simulink model "PubIfDecisionTOS_MDL"  (R2020b)
settings: configuration reference "DspaceConfig" (kept outside this file)
PostLoadFcn:
  | if any(exist('dsrtsu_mdlpostloadfcn', 'file') ~= 0), dsrtsu_mdlpostloadfcn('Execute', bdroot); end
InitFcn:
  | , if any(exist('dsmpb_private', 'file') ~= 0), dsmpb_private('dsmpb_mdlclblib', 'Init', bdroot); end,
undefined symbols (not defined in the file or in its folder): C_TOS_ACCEgoRAxletoFbumplength_m, C_TOS_ACCTargetFront_Flag, C_TOS_AEBJAPedObjDxThre_Val, C_TOS_AEBJAPedObjDyThre_Val, C_TOS_AEBJATargetSize_Val, C_TOS_AEBJAVehObjDxThre_Val, C_TOS_AEBJAVehObjDyThre_Val, C_TOS_AEBJuncPedTargetSize_Val, C_TOS_AEBLatObjDxThre_Val, C_TOS_AEBLatPedDyThre_Val, C_TOS_AEBLatTargetSize_Val, C_TOS_AEBLongTargetInEgoFront_Flag, C_TOS_axAbsGround_Parameter, C_TOS_CameraConfirmedFlag, C_TOS_CNsubjWidth, C_TOS_CurrentLaneCoreMinWidth_Val, C_TOS_CutInProb_Val_Zero, C_TOS_CutOutProb_Val_Zero, C_TOS_D2R_Val, C_TOS_DefaultValueObjectToCenterLine_dy, C_TOS_EgoCarWidth_Val, C_TOS_EgoDxRefPoint_m, C_TOS_EgoRAxletoFbumplength_m, C_TOS_HalfWidthVehicle_Con, C_TOS_HWA_CurrentLaneFlag, C_TOS_HWA_LeftLaneFlag, C_TOS_HWA_MovingDir_Vaild, C_TOS_HWA_MovState_Vaild, C_TOS_HWA_RightLaneFlag, C_TOS_LaneLineCourseErrorFront, C_TOS_LaneLineCourseErrorRear, C_TOS_MotorbikeDefaultWidth_m, C_TOS_NumberOfEffectiveTargets, C_TOS_Obj_Age_Val, C_TOS_Objdx_Constraint_Val, C_TOS_ObjectDefaultWidth_m, C_TOS_ObjInCurrentLane_Val, C_TOS_ObjInCurrentLaneValid, C_TOS_ObjInLeftLaneValid, C_TOS_ObjInRightLaneValid, C_TOS_ObjNotInCurrentLane_Val, C_TOS_ObjNotREElementType, C_TOS_ObjPredictDis_dy_ConstantVal_Zeros, C_TOS_ObjToCenterLine_ConstantVal_Zeros, C_TOS_OFMObjIDInvilad_Val, C_TOS_PIL_LatDisCons_Val_zero, C_TOS_PIL_ObjectCutInFlag_b, C_TOS_PIL_ObjectCutOutFlag_b, C_TOS_PIL_ObjLaneProb_al_Val, C_TOS_PP_ObjFusType_FC_Confirm_b, C_TOS_PP_ObjFusType_FC_FR_Confirm_b, C_TOS_PP_ObjFusType_FR_Confirm_b, C_TOS_RE_80BoolDefault_Val, C_TOS_RE_80Single181Default_Val, C_TOS_RE_80Single255Default_Val, C_TOS_RE_80Uint8Default_Val, C_TOS_RE_D2R, C_TOS_RE_D_180_Val, C_TOS_RE_InvalidObjectID_Val, C_TOS_RE_InvalidTargetChainDir_Val ... (+142)
libraries: simulink x1650, TOS_LIB x361, canfdmsglib x14
(part 51 of 69)

== system PubIfDecisionTOS_MDL/TOS_20201112/TOS_2012080320/TOS/ACC/TOS_ACCCurrentLane/ACC_CurrentLane_Target/TOS_ACC_P0/ACC_P0_Targe/ACC_P0_Targe/TOS_ACC_ObstacleProbConfirm/TOS_ACCObstacleProbAborDly ==
  ACC_Target_ID_K1 : Inport
  ObjectID : Inport  Port=2
  TOS_ACCObstacleProb : Inport  Port=3
  If : If  IfExpression=u1
  If Action Subsystem : Subsystem  TreatAsAtomicUnit=on
  If Action Subsystem1 : Subsystem  TreatAsAtomicUnit=on
  Merge : Merge
  Subsystem : Subsystem
  TOS_ACCObstacleProbFilt : Outport
  wires:
  If/1 -> If Action Subsystem1/Action
  TOS_ACCObstacleProb/1 -> If Action Subsystem1/1(TOS_ACCFusionType), If Action Subsystem/1(TOS_ACCFusionType)
  If/2 -> If Action Subsystem/Action
  ACC_Target_ID_K1/1 -> Subsystem/1(ACC_TargetP0_ID_K1)
  ObjectID/1 -> Subsystem/2(ObjectID)
  Subsystem/1(ACC_SameTargetP0) -> If/1
  If Action Subsystem1/1(TOS_ACCFusionTypeFilt) -> Merge/1
  If Action Subsystem/1(TOS_ACCFusionTypeFilt) -> Merge/2
  Merge/1 -> TOS_ACCObstacleProbFilt/1

== system PubIfDecisionTOS_MDL/TOS_20201112/TOS_2012080320/TOS/ACC/TOS_ACCCurrentLane/ACC_CurrentLane_Target/TOS_ACC_P0/ACC_P0_Targe/ACC_P0_Targe/TOS_ACC_TargetMovingDirConfirm/Subsystem ==
  ObjMovState : Inport
  ACC_Target_ID_K1 : Inport  Port=2
  ACC_Target_ID_K2 : Inport  Port=3
  ACC_Target_MovState_K1 : Inport  Port=4
  ACC_Target_MovState_K2 : Inport  Port=5
  ObjectID : Inport  Port=6
  TOS_ObjMovStateCfmFlow : Stateflow chart  TreatAsAtomicUnit=on
  TOS_ObjMovStateCfm : Outport
  wires:
  TOS_ObjMovStateCfmFlow/1(TOS_ObjMovStateCfm) -> TOS_ObjMovStateCfm/1
  ACC_Target_ID_K1/1 -> TOS_ObjMovStateCfmFlow/1(Target_ID_K1)
  ACC_Target_ID_K2/1 -> TOS_ObjMovStateCfmFlow/2(Target_ID_K2)
  ACC_Target_MovState_K1/1 -> TOS_ObjMovStateCfmFlow/3(Target_MovState_K1)
  ACC_Target_MovState_K2/1 -> TOS_ObjMovStateCfmFlow/4(Target_MovState_K2)
  ObjMovState/1 -> TOS_ObjMovStateCfmFlow/5(ObjMovState)
  ObjectID/1 -> TOS_ObjMovStateCfmFlow/6(ObjectID)

== system PubIfDecisionTOS_MDL/TOS_20201112/TOS_2012080320/TOS/ACC/TOS_ACCCurrentLane/ACC_CurrentLane_Target/TOS_ACC_P0/ACC_P0_Targe/ACC_P0_Targe/TOS_ACC_TargetMovingDirConfirm/TOS_ACCMovingDirAborDly ==
  ACC_TargetP0_ID_K1 : Inport
  ObjectID : Inport  Port=2
  TOS_ACCMovingDir : Inport  Port=3
  If : If  IfExpression=u1
  If Action Subsystem : Subsystem  TreatAsAtomicUnit=on
  If Action Subsystem1 : Subsystem  TreatAsAtomicUnit=on
  Merge : Merge
  Subsystem : Subsystem
  TOS_ACC_TrgMovDirFlag_6_ObserVale : Outport
  TOS_ACC_TrgMovDir : Outport  Port=2
  wires:
  If/1 -> If Action Subsystem1/Action
  TOS_ACCMovingDir/1 -> If Action Subsystem1/1(TOS_ACCMovingDir), If Action Subsystem/1(TOS_ACCMovingDir)
  If/2 -> If Action Subsystem/Action
  ACC_TargetP0_ID_K1/1 -> Subsystem/1(ACC_TargetP0_ID_K1)
  ObjectID/1 -> Subsystem/2(ObjectID)
  Subsystem/1(ACC_SameTargetP0) -> TOS_ACC_TrgMovDirFlag_6_ObserVale/1, If/1
  If Action Subsystem1/1(TOS_ACCMovingDirFilt) -> Merge/1
  If Action Subsystem/1(TOS_ACCMovingDirFilt) -> Merge/2
  Merge/1 -> TOS_ACC_TrgMovDir/1

== system PubIfDecisionTOS_MDL/TOS_20201112/TOS_2012080320/TOS/ACC/TOS_ACCCurrentLane/ACC_CurrentLane_Target/TOS_ACC_P0/ACC_P0_Targe/ACC_P0_Targe/TOS_ACC_TargetMovingDirConfirm/TOS_ACC_TargetMovingDirConfirm_V2011170316(备份) ==
  note: 已选中目标，前两个周期为运动，以后为运动，前两个周期为Stopped，以后为Stopped
  note: 去除横穿目标
  object_MovingState : Inport
  PP_ObjMovingDirSignalProcessing : Inport  Port=2
  Object_HeadingAngle : Inport  Port=3
  Object_VX : Inport  Port=4
  Object_VY : Inport  Port=5
  VIE_EgoVelocity : Inport  Port=6
  SteerWheelAng : Inport  Port=7
  ACC_Target_ID_K1 : Inport  Port=8
  ACC_Target_ID_K2 : Inport  Port=9
  ACC_Target_MovState_K1 : Inport  Port=10
  ACC_Target_MovState_K2 : Inport  Port=11
  ObjectID : Inport  Port=12
  Abs{,1..4} (5 alike) : Abs
  Add : Sum
  Compare To Constant : simulink/Logic and Bit Operations/Compare To Constant  relop===  const=ObjectMovingOrientation_E.SameDir  OutDataTypeStr=boolean
      settings: AttributesFormatString=ObjectMovingOrientation_E.SameDir = 1
  Compare To Constant1 : simulink/Logic and Bit Operations/Compare To Constant  relop===  const=OFM_OBJ_MOVINGSTATE_E.MOVING  OutDataTypeStr=boolean
      settings: AttributesFormatString=OFM_OBJ_MOVINGSTATE_E.MOVING = 2
  Compare To Constant10 : simulink/Logic and Bit Operations/Compare To Constant  relop=<=  const=P_TOS_ObjLatCroYawAngMaxThre_Val  OutDataTypeStr=boolean
      settings: AttributesFormatString=P_TOS_ObjLatCroYawAngMaxThre_Val = 135
  Compare To Constant11 : simulink/Logic and Bit Operations/Compare To Constant  relop===  const=1  OutDataTypeStr=boolean
  Compare To Constant12 : simulink/Logic and Bit Operations/Compare To Constant  relop===  const=2  OutDataTypeStr=boolean
  Compare To Constant13 : simulink/Logic and Bit Operations/Compare To Constant  relop=<  const=1.5  OutDataTypeStr=boolean
      settings: AttributesFormatString=1.5 m/s
  Compare To Constant2 : simulink/Logic and Bit Operations/Compare To Constant  relop=>=  const=P_TOS_ObjInSameDirYawAngMinThre_Val  OutDataTypeStr=boolean
      settings: AttributesFormatString=P_TOS_ObjInSameDirYawAngMinThre_Val = 0
  Compare To Constant3 : simulink/Logic and Bit Operations/Compare To Constant  relop=<=  const=P_TOS_ObjInSameDirYawAngMaxThre_Val  OutDataTypeStr=boolean
      settings: AttributesFormatString=P_TOS_ObjInSameDirYawAngMaxThre_Val = 45
  Compare To Constant4 : simulink/Logic and Bit Operations/Compare To Constant  relop===  const=OFM_OBJ_MOVINGSTATE_E.MOVING_SLOWLY  OutDataTypeStr=boolean
      settings: AttributesFormatString=OFM_OBJ_MOVINGSTATE_E.MOVING_SLOWLY = 5
  Compare To Constant5 : simulink/Logic and Bit Operations/Compare To Constant  relop=<  const=P_TOS_SameDirVyOffset_Val  OutDataTypeStr=boolean
      settings: AttributesFormatString=P_TOS_SameDirVyOffset_Val = 2
  Compare To Constant6 : simulink/Logic and Bit Operations/Compare To Constant  relop===  const=ObjectMovingOrientation_E.Crossing  OutDataTypeStr=boolean
      settings: AttributesFormatString=ObjectMovingOrientation_E.Crossing = 3
  Compare To Constant7 : simulink/Logic and Bit Operations/Compare To Constant  relop=>=  const=P_TOS_LongVyThre_Val  OutDataTypeStr=boolean
      settings: AttributesFormatString=P_TOS_LongVyThre_Val = 2
  Compare To Constant8 : simulink/Logic and Bit Operations/Compare To Constant  relop===  const=OFM_OBJ_MOVINGSTATE_E.STOPPED  OutDataTypeStr=boolean
      settings: AttributesFormatString=OFM_OBJ_MOVINGSTATE_E.STOPPED = 4
  Compare To Constant9 : simulink/Logic and Bit Operations/Compare To Constant  relop=>=  const=P_TOS_ObjInSameDirYawAngMaxThre_Val  OutDataTypeStr=boolean
      settings: AttributesFormatString=P_TOS_ObjInSameDirYawAngMaxThre_Val = 45
  Constant1 : Constant  Value=P_TOS_SameDirVxvOffset_Val
      settings: AttributesFormatString=P_TOS_AEBLong_SameDirVxvOffset_Val = 1
  Constant2 : Constant  Value=0  OutDataTypeStr=boolean
  Constant3 : Constant  OutDataTypeStr=boolean
  Constant4 : Constant  OutDataTypeStr=boolean
  Data Type Conversion1 : DataTypeConversion  OutDataTypeStr=Enum: ObjectMovingOrientation_E
  Data Type Conversion2 : DataTypeConversion  OutDataTypeStr=Enum: OFM_OBJ_MOVINGSTATE_E
  Logical Operator{,3,6,8} (4 alike) : Logic  AllPortsSameDT=off  OutDataTypeStr=boolean
  Logical Operator{1,4..5,7} (4 alike) : Logic  Operator=OR  AllPortsSameDT=off  OutDataTypeStr=boolean
  Logical Operator2 : Logic  Operator=OR  Inputs=3  AllPortsSameDT=off  OutDataTypeStr=boolean
  Relational Operator : RelationalOperator  Operator=<  OutDataTypeStr=boolean  RndMeth=Simplest
  Subsystem : Subsystem
  Switch : Switch  Criteria=u2 > Threshold
  Switch1 : Switch  Criteria=u2 ~= 0
  Switch2 : Switch  Criteria=u2 ~= 0
  TOS_ACCMovingDirAborDly : Subsystem
  Terminator : Terminator
  Terminator1 : Terminator
  TOS_ACC_TrgMovDir : Outport
  TOS_ACC_TrgMovDirFlag_1_ObserVale : Outport  Port=2
  TOS_ACC_TrgMovDirFlag_2_ObserVale : Outport  Port=3
  TOS_ACC_TrgMovDirFlag_3_ObserVale : Outport  Port=4
  TOS_ACC_TrgMovDirFlag_4_ObserVale : Outport  Port=5
  TOS_ACC_TrgMovDirFlag_5_ObserVale : Outport  Port=6
  TOS_ACC_TrgMovDirFlag_6_ObserVale : Outport  Port=7
  wires:
  Compare To Constant13/1 -> Logical Operator8/2
  Abs3/1 -> Compare To Constant13/1
  [Object_VY] -> Abs3/1
  Constant4/1 -> Logical Operator8/1
  TOS_ACCMovingDirAborDly/2(TOS_ACC_TrgMovDir) -> TOS_ACC_TrgMovDir/1
  TOS_ACCMovingDirAborDly/1(TOS_ACC_TrgMovDirFlag_6_ObserVale) -> [TOS_ACC_TrgMovDirFlag_6_ObserVale]
  [TOS_ACC_TrgMovDirFlag_6_ObserVale] -> TOS_ACC_TrgMovDirFlag_6_ObserVale/1
  [TOS_ACC_TrgMovDirFlag_5_ObserVale] -> TOS_ACC_TrgMovDirFlag_5_ObserVale/1
  [TOS_ACC_TrgMovDirFlag_4_ObserVale] -> TOS_ACC_TrgMovDirFlag_4_ObserVale/1
  [TOS_ACC_TrgMovDirFlag_3_ObserVale] -> TOS_ACC_TrgMovDirFlag_3_ObserVale/1
  [TOS_ACC_TrgMovDirFlag_2_ObserVale] -> TOS_ACC_TrgMovDirFlag_2_ObserVale/1
  [TOS_ACC_TrgMovDirFlag_1_ObserVale] -> TOS_ACC_TrgMovDirFlag_1_ObserVale/1
  Logical Operator7/1 -> Switch2/2, [TOS_ACC_TrgMovDirFlag_3_ObserVale]
  Compare To Constant12/1 -> Logical Operator7/1
  ACC_Target_ID_K1/1 -> Subsystem/2(ACC_Target_ID_K1), [ACC_Target_ID_K1]
  ACC_Target_MovState_K1/1 -> Subsystem/4(ACC_Target_MovState_K1)
  ACC_Target_ID_K2/1 -> Subsystem/3(ACC_Target_ID_K2)
  ACC_Target_MovState_K2/1 -> Subsystem/5(ACC_Target_MovState_K2)
  Data Type Conversion2/1 -> Compare To Constant4/1, Subsystem/1(ObjMovState), Compare To Constant8/1, Compare To Constant1/1
  Subsystem/1(TOS_ObjMovStateCfm) -> Compare To Constant12/1, Compare To Constant11/1
  Compare To Constant11/1 -> Logical Operator2/3
  ObjectID/1 -> Subsystem/6(ObjectID), [ObjectID]
  Logical Operator8/1 -> Switch2/1
  Switch2/1 -> Switch/3
  Compare To Constant8/1 -> Logical Operator7/2
  Switch1/1 -> Switch2/3
  Logical Operator6/1 -> Logical Operator5/2
  Compare To Constant10/1 -> Logical Operator6/2
  Compare To Constant9/1 -> Logical Operator6/1
  [Object_HeadingAngle] -> Compare To Constant9/1, Compare To Constant10/1
  Compare To Constant6/1 -> Logical Operator5/1
  [PP_ObjMovingDirSignalProcessing] -> Compare To Constant6/1
  Switch/1 -> TOS_ACCMovingDirAborDly/3(TOS_ACCMovingDir), [TOS_ACC_TrgMovDirFlag_5_ObserVale]
  [ObjectID] -> TOS_ACCMovingDirAborDly/2(ObjectID)
  [ACC_Target_ID_K1] -> TOS_ACCMovingDirAborDly/1(ACC_TargetP0_ID_K1)
  Abs4/1 -> Compare To Constant7/1
  [Object_VY] -> Abs4/1
  Logical Operator5/1 -> Logical Operator4/1
  Compare To Constant7/1 -> Logical Operator4/2
  Constant2/1 -> Switch1/1
  Logical Operator4/1 -> Switch1/2, [TOS_ACC_TrgMovDirFlag_4_ObserVale]
  Constant3/1 -> Switch1/3
  SteerWheelAng/1 -> Terminator/1
  Abs2/1 -> Compare To Constant5/1
  Object_VY/1 -> Abs2/1, [Object_VY]
  Object_VX/1 -> Abs1/1
  VIE_EgoVelocity/1 -> Relational Operator/2
  Add/1 -> Relational Operator/1
  Constant1/1 -> Add/2
  Abs1/1 -> Add/1
  Relational Operator/1 -> Logical Operator/1
  Compare To Constant5/1 -> Logical Operator/2
  Logical Operator/1 -> Logical Operator1/2
  Abs/1 -> [Object_HeadingAngle], Compare To Constant3/1, Compare To Constant2/1
  PP_ObjMovingDirSignalProcessing/1 -> Data Type Conversion1/1
  Logical Operator1/1 -> [TOS_ACC_TrgMovDirFlag_1_ObserVale], Switch/1
  Data Type Conversion1/1 -> [PP_ObjMovingDirSignalProcessing], Compare To Constant/1
  Compare To Constant2/1 -> Logical Operator3/1
  Compare To Constant3/1 -> Logical Operator3/2
  Object_HeadingAngle/1 -> Abs/1
  Compare To Constant/1 -> Logical Operator1/1
  Logical Operator3/1 -> Terminator1/1
  object_MovingState/1 -> Data Type Conversion2/1
  Compare To Constant4/1 -> Logical Operator2/2
  Compare To Constant1/1 -> Logical Operator2/1
  Logical Operator2/1 -> Switch/2, [TOS_ACC_TrgMovDirFlag_2_ObserVale]

== system PubIfDecisionTOS_MDL/TOS_20201112/TOS_2012080320/TOS/ACC/TOS_ACCCurrentLane/ACC_CurrentLane_Target/TOS_ACC_P1/ACC_P1_Targe/ACC_P1_Targe/TOS_ACC_DyConfirm/OverLapConfirm ==
  DyConfirm_Sig : Inport
  Abs{,1..4} (5 alike) : Abs
  Bus Creator{1..4} (4 alike) : BusCreator  Inputs=2
  Bus Selector : BusSelector  OutputSignals=PositionFlag,Line_pC2
  Bus Selector1 : BusSelector  OutputSignals=PositionFlag,Line_pC2
  Bus Selector2 : BusSelector  OutputSignals=LM_LR_Line04_pC0,LM_RL_Line04_pC0
  Bus Selector3 : BusSelector  OutputSignals=PositionFlag,Line_pC2
  Bus Selector4 : BusSelector  OutputSignals=LM_LR_Line04_pC2,Object_DX,LM_LR_Line04_dDisStart,LM_LR_Line04_dDisEnd,LM_LR_Line04_fCamValid
  Bus Selector5 : BusSelector  OutputSignals=LM_LR_Line05_pC2,Object_DX,LM_LR_Line05_dDisStart,LM_LR_Line05_dDisEnd,LM_LR_Line05_fCamValid
  Bus Selector8 : BusSelector  OutputSignals=LM_LR_Line06_pC2,Object_DX,LM_LR_Line06_dDisStart,LM_LR_Line06_dDisEnd,LM_LR_Line06_fCamValid
  Compare To Constant : simulink/Logic and Bit Operations/Compare To Constant  relop===  const=uint8(4)  OutDataTypeStr=boolean
  Compare To Constant1 : simulink/Logic and Bit Operations/Compare To Constant  relop=>=  const=single(0.001)  OutDataTypeStr=boolean
  Compare To Constant2 : simulink/Logic and Bit Operations/Compare To Constant  relop=>=  const=single(0.001)  OutDataTypeStr=boolean
  Compare To Constant3 : simulink/Logic and Bit Operations/Compare To Constant  relop===  const=uint8(5)  OutDataTypeStr=boolean
  Compare To Constant4 : simulink/Logic and Bit Operations/Compare To Constant  relop=>=  const=single(0.001)  OutDataTypeStr=boolean
  Compare To Constant5 : simulink/Logic and Bit Operations/Compare To Constant  relop===  const=uint8(6)  OutDataTypeStr=boolean
  Constant : Constant  Value=0  OutDataTypeStr=uint8
  Constant1 : Constant  Value=4  OutDataTypeStr=uint8
  Constant2 : Constant  Value=5  OutDataTypeStr=uint8
  Constant3 : Constant  Value=6  OutDataTypeStr=uint8
  Constant4 : Constant  Value=0  OutDataTypeStr=single
  Logical Operator1 : Logic  AllPortsSameDT=off  OutDataTypeStr=boolean
  Logical Operator10 : Logic  Inputs=3  AllPortsSameDT=off  OutDataTypeStr=boolean
  Logical Operator11 : Logic  Inputs=3  AllPortsSameDT=off  OutDataTypeStr=boolean
  Logical Operator2 : Logic  AllPortsSameDT=off  OutDataTypeStr=boolean
  Logical Operator3 : Logic  AllPortsSameDT=off  OutDataTypeStr=boolean
  Logical Operator4 : Logic  Operator=OR  Inputs=3  AllPortsSameDT=off  OutDataTypeStr=boolean
  Logical Operator5 : Logic  Operator=OR  AllPortsSameDT=off  OutDataTypeStr=boolean
  Logical Operator6 : Logic  Operator=OR  AllPortsSameDT=off  OutDataTypeStr=boolean
  Logical Operator7 : Logic  Operator=OR  AllPortsSameDT=off  OutDataTypeStr=boolean
  Logical Operator9 : Logic  Inputs=3  AllPortsSameDT=off  OutDataTypeStr=boolean
  Relational Operator : RelationalOperator  Operator=~=  OutDataTypeStr=boolean  RndMeth=Simplest
  Relational Operator4 : RelationalOperator  Operator=>  OutDataTypeStr=boolean  RndMeth=Simplest
  Relational Operator5 : RelationalOperator  Operator=<=  OutDataTypeStr=boolean  RndMeth=Simplest
  Relational Operator6 : RelationalOperator  Operator=>  OutDataTypeStr=boolean  RndMeth=Simplest
  Relational Operator7 : RelationalOperator  Operator=<=  OutDataTypeStr=boolean  RndMeth=Simplest
  Relational Operator8 : RelationalOperator  Operator=>  OutDataTypeStr=boolean  RndMeth=Simplest
  Relational Operator9 : RelationalOperator  Operator=<=  OutDataTypeStr=boolean  RndMeth=Simplest
  Signal Copy : SignalConversion  OverrideOpt=off
  Signal Copy1 : SignalConversion  OverrideOpt=off
  Signal Copy2 : SignalConversion  OverrideOpt=off
  Switch3 : Switch  Criteria=u2 > Threshold  OutDataTypeStr=single
  Switch4 : Switch  Criteria=u2 > Threshold  OutDataTypeStr=single
  Switch5 : Switch  Criteria=u2 > Threshold  OutDataTypeStr=single
  TOS_ACC_OverlapRatio : Outport
  wires:
  Logical Operator7/1 -> Logical Operator11/3
  [C0_Confirm] -> Logical Operator7/2
  Logical Operator6/1 -> Logical Operator10/3
  [C0_Confirm] -> Logical Operator6/2
  Logical Operator5/1 -> Logical Operator9/3
  [C0_Confirm] -> Logical Operator5/2
  Relational Operator/1 -> [C0_Confirm]
  Abs4/1 -> Relational Operator/2
  Abs3/1 -> Relational Operator/1
  Bus Selector2/2 -> Abs4/1  "<LM_RL_Line04_pC0>"
  Bus Selector2/1 -> Abs3/1  "<LM_LR_Line04_pC0>"
  Abs2/1 -> Compare To Constant4/1
  Abs1/1 -> Compare To Constant2/1
  Abs/1 -> Compare To Constant1/1
  Logical Operator4/1 -> TOS_ACC_OverlapRatio/1
  Logical Operator3/1 -> Logical Operator4/3
  Logical Operator2/1 -> Logical Operator4/2
  Bus Selector3/2 -> Abs2/1  "<Line_pC2>"
  Bus Selector3/1 -> Compare To Constant5/1  "<PositionFlag>"
  Switch3/1 -> Bus Selector/1, Bus Selector1/1, Bus Selector3/1
  Compare To Constant5/1 -> Logical Operator3/1
  Compare To Constant4/1 -> Logical Operator3/2
  Compare To Constant2/1 -> Logical Operator2/2
  Compare To Constant3/1 -> Logical Operator2/1
  Bus Selector1/1 -> Compare To Constant3/1  "<PositionFlag>"
  Bus Selector1/2 -> Abs1/1  "<Line_pC2>"
  Logical Operator1/1 -> Logical Operator4/1
  Compare To Constant1/1 -> Logical Operator1/2
  DyConfirm_Sig/1 -> Bus Selector2/1, Bus Selector4/1, Bus Selector5/1, Bus Selector8/1
  Compare To Constant/1 -> Logical Operator1/1
  Bus Selector/2 -> Abs/1  "<Line_pC2>"
  Bus Selector/1 -> Compare To Constant/1  "<PositionFlag>"
  Constant4/1 -> Bus Creator4/2  "Line_pC2"
  Bus Creator3/1 -> Switch5/1
  Signal Copy2/1 -> Bus Creator3/2  "Line_pC2"
  Bus Selector4/1 -> Signal Copy/1  "<LM_LR_Line04_pC2>"
  Logical Operator9/1 -> Switch3/2
  Bus Selector5/1 -> Signal Copy1/1  "<LM_LR_Line05_pC2>"
  Constant/1 -> Bus Creator4/1  "PositionFlag"
  Signal Copy1/1 -> Bus Creator2/2  "Line_pC2"
  Constant3/1 -> Bus Creator3/1  "PositionFlag"
  Constant2/1 -> Bus Creator2/1  "PositionFlag"
  Bus Selector4/4 -> Relational Operator5/2  "<LM_LR_Line04_dDisEnd>"
  Bus Creator4/1 -> Switch5/3
  Relational Operator7/1 -> Logical Operator10/2
  Relational Operator6/1 -> Logical Operator10/1
  Constant1/1 -> Bus Creator1/1  "PositionFlag"
  Relational Operator4/1 -> Logical Operator9/1
  Bus Creator2/1 -> Switch4/1
  Bus Selector5/5 -> Logical Operator6/1  "<LM_LR_Line05_fCamValid>"
  Switch5/1 -> Switch4/3
  Bus Selector8/5 -> Logical Operator7/1  "<LM_LR_Line06_fCamValid>"
  Bus Selector5/2 -> Relational Operator7/1, Relational Operator6/1  "<Object_DX>"
  Bus Selector5/3 -> Relational Operator6/2  "<LM_LR_Line05_dDisStart>"
  Logical Operator11/1 -> Switch5/2
  Bus Creator1/1 -> Switch3/1
  Bus Selector8/4 -> Relational Operator9/2  "<LM_LR_Line06_dDisEnd>"
  Switch4/1 -> Switch3/3
  Relational Operator9/1 -> Logical Operator11/2
  Bus Selector8/1 -> Signal Copy2/1  "<LM_LR_Line06_pC2>"
  Bus Selector8/3 -> Relational Operator8/2  "<LM_LR_Line06_dDisStart>"
  Signal Copy/1 -> Bus Creator1/2  "Line_pC2"
  Relational Operator5/1 -> Logical Operator9/2
  Relational Operator8/1 -> Logical Operator11/1
  Bus Selector4/2 -> Relational Operator4/1, Relational Operator5/1  "<Object_DX>"
  Bus Selector5/4 -> Relational Operator7/2  "<LM_LR_Line05_dDisEnd>"
  Bus Selector4/3 -> Relational Operator4/2  "<LM_LR_Line04_dDisStart>"
  Bus Selector4/5 -> Logical Operator5/1  "<LM_LR_Line04_fCamValid>"
  Bus Selector8/2 -> Relational Operator8/1, Relational Operator9/1  "<Object_DX>"
  Logical Operator10/1 -> Switch4/2

== system PubIfDecisionTOS_MDL/TOS_20201112/TOS_2012080320/TOS/ACC/TOS_ACCCurrentLane/ACC_CurrentLane_Target/TOS_ACC_P1/ACC_P1_Targe/ACC_P1_Targe/TOS_ACC_FusionTypeConfirm/Subsystem1 ==
  ObjMovState : Inport
  ACC_Target_ID_K1 : Inport  Port=2
  ACC_Target_ID_K2 : Inport  Port=3
  ACC_Target_MovState_K1 : Inport  Port=4
  ACC_Target_MovState_K2 : Inport  Port=5
  ObjectID : Inport  Port=6
  TOS_ObjMovStateCfmFlow1 : Stateflow chart  TreatAsAtomicUnit=on
  TOS_ObjMovStateCfm : Outport
  wires:
  ObjectID/1 -> TOS_ObjMovStateCfmFlow1/6(ObjectID)
  ObjMovState/1 -> TOS_ObjMovStateCfmFlow1/5(ObjMovState)
  ACC_Target_MovState_K2/1 -> TOS_ObjMovStateCfmFlow1/4(Target_MovState_K2)
  ACC_Target_MovState_K1/1 -> TOS_ObjMovStateCfmFlow1/3(Target_MovState_K1)
  ACC_Target_ID_K2/1 -> TOS_ObjMovStateCfmFlow1/2(Target_ID_K2)
  ACC_Target_ID_K1/1 -> TOS_ObjMovStateCfmFlow1/1(Target_ID_K1)
  TOS_ObjMovStateCfmFlow1/1(TOS_ObjMovStateCfm) -> TOS_ObjMovStateCfm/1

== system PubIfDecisionTOS_MDL/TOS_20201112/TOS_2012080320/TOS/ACC/TOS_ACCCurrentLane/ACC_CurrentLane_Target/TOS_ACC_P1/ACC_P1_Targe/ACC_P1_Targe/TOS_ACC_FusionTypeConfirm/TOS_ACCFusionTypeAborDly ==
  ACC_TargetP0_ID_K1 : Inport
  ObjectID : Inport  Port=2
  TOS_ACCFusionType : Inport  Port=3
  If : If  IfExpression=u1
  If Action Subsystem : Subsystem  TreatAsAtomicUnit=on
  If Action Subsystem1 : Subsystem  TreatAsAtomicUnit=on
  Merge : Merge
  Relational Operator : RelationalOperator  Operator===  OutDataTypeStr=boolean  RndMeth=Simplest
  TOS_ACCFusionTypeFilt : Outport
  wires:
  Merge/1 -> TOS_ACCFusionTypeFilt/1
  If Action Subsystem/1(TOS_ACCFusionTypeFilt) -> Merge/2
  If Action Subsystem1/1(TOS_ACCFusionTypeFilt) -> Merge/1
  Relational Operator/1 -> If/1
  ObjectID/1 -> Relational Operator/2
  ACC_TargetP0_ID_K1/1 -> Relational Operator/1
  If/2 -> If Action Subsystem/Action
  TOS_ACCFusionType/1 -> If Action Subsystem/1(TOS_ACCFusionType), If Action Subsystem1/1(TOS_ACCFusionType)
  If/1 -> If Action Subsystem1/Action

== system PubIfDecisionTOS_MDL/TOS_20201112/TOS_2012080320/TOS/ACC/TOS_ACCCurrentLane/ACC_CurrentLane_Target/TOS_ACC_P1/ACC_P1_Targe/ACC_P1_Targe/TOS_ACC_ObjTypeConfirm/Subsystem ==
  ObjMovState : Inport
  ACC_Target_ID_K1 : Inport  Port=2
  ACC_Target_ID_K2 : Inport  Port=3
  ACC_Target_MovState_K1 : Inport  Port=4
  ACC_Target_MovState_K2 : Inport  Port=5
  ObjectID : Inport  Port=6
  TOS_ObjMovStateCfmFlow1 : Stateflow chart  TreatAsAtomicUnit=on
  TOS_ObjMovStateCfm : Outport
  wires:
  ObjectID/1 -> TOS_ObjMovStateCfmFlow1/6(ObjectID)
  ObjMovState/1 -> TOS_ObjMovStateCfmFlow1/5(ObjMovState)
  ACC_Target_MovState_K2/1 -> TOS_ObjMovStateCfmFlow1/4(ACC_TargetP0_MovState_K2)
  ACC_Target_MovState_K1/1 -> TOS_ObjMovStateCfmFlow1/3(ACC_TargetP0_MovState_K1)
  ACC_Target_ID_K2/1 -> TOS_ObjMovStateCfmFlow1/2(ACC_TargetP0_ID_K2)
  ACC_Target_ID_K1/1 -> TOS_ObjMovStateCfmFlow1/1(ACC_TargetP0_ID_K1)
  TOS_ObjMovStateCfmFlow1/1(TOS_ObjMovStateCfm) -> TOS_ObjMovStateCfm/1

== system PubIfDecisionTOS_MDL/TOS_20201112/TOS_2012080320/TOS/ACC/TOS_ACCCurrentLane/ACC_CurrentLane_Target/TOS_ACC_P1/ACC_P1_Targe/ACC_P1_Targe/TOS_ACC_ObjTypeConfirm/TOS_ACCObjTypeAborDly ==
  ACC_Target_ID_K1 : Inport
  ObjectID : Inport  Port=2
  TOS_ACCObjType : Inport  Port=3
  If : If  IfExpression=u1
  If Action Subsystem : Subsystem  TreatAsAtomicUnit=on
  If Action Subsystem1 : Subsystem  TreatAsAtomicUnit=on
  Merge : Merge
  Relational Operator : RelationalOperator  Operator===  OutDataTypeStr=boolean  RndMeth=Simplest
  TOS_ACCObjTypeFilt : Outport
  wires:
  Merge/1 -> TOS_ACCObjTypeFilt/1
  If Action Subsystem/1(TOS_ACCFusionTypeFilt) -> Merge/2
  If Action Subsystem1/1(TOS_ACCFusionTypeFilt) -> Merge/1
  Relational Operator/1 -> If/1
  ObjectID/1 -> Relational Operator/2
  ACC_Target_ID_K1/1 -> Relational Operator/1
  If/2 -> If Action Subsystem/Action
  TOS_ACCObjType/1 -> If Action Subsystem/1(TOS_ACCFusionType), If Action Subsystem1/1(TOS_ACCFusionType)
  If/1 -> If Action Subsystem1/Action

== system PubIfDecisionTOS_MDL/TOS_20201112/TOS_2012080320/TOS/ACC/TOS_ACCCurrentLane/ACC_CurrentLane_Target/TOS_ACC_P1/ACC_P1_Targe/ACC_P1_Targe/TOS_ACC_ObstacleProbConfirm/TOS_ACCObstacleProbAborDly ==
  ACC_Target_ID_K1 : Inport
  ObjectID : Inport  Port=2
  TOS_ACCObstacleProb : Inport  Port=3
  If : If  IfExpression=u1
  If Action Subsystem : Subsystem  TreatAsAtomicUnit=on
  If Action Subsystem1 : Subsystem  TreatAsAtomicUnit=on
  Merge : Merge
  Subsystem : Subsystem
  TOS_ACCObstacleProbFilt : Outport
  wires:
  Merge/1 -> TOS_ACCObstacleProbFilt/1
  If Action Subsystem/1(TOS_ACCFusionTypeFilt) -> Merge/2
  If Action Subsystem1/1(TOS_ACCFusionTypeFilt) -> Merge/1
  Subsystem/1(ACC_SameTargetP0) -> If/1
  ObjectID/1 -> Subsystem/2(ObjectID)
  ACC_Target_ID_K1/1 -> Subsystem/1(ACC_TargetP0_ID_K1)
  If/2 -> If Action Subsystem/Action
  TOS_ACCObstacleProb/1 -> If Action Subsystem/1(TOS_ACCFusionType), If Action Subsystem1/1(TOS_ACCFusionType)
  If/1 -> If Action Subsystem1/Action

== system PubIfDecisionTOS_MDL/TOS_20201112/TOS_2012080320/TOS/ACC/TOS_ACCCurrentLane/ACC_CurrentLane_Target/TOS_ACC_P1/ACC_P1_Targe/ACC_P1_Targe/TOS_ACC_TargetMovingDirConfirm/Subsystem ==
  ObjMovState : Inport
  ACC_Target_ID_K1 : Inport  Port=2
  ACC_Target_ID_K2 : Inport  Port=3
  ACC_Target_MovState_K1 : Inport  Port=4
  ACC_Target_MovState_K2 : Inport  Port=5
  ObjectID : Inport  Port=6
  TOS_ObjMovStateCfmFlow : Stateflow chart  TreatAsAtomicUnit=on
  TOS_ObjMovStateCfm : Outport
  wires:
  ObjectID/1 -> TOS_ObjMovStateCfmFlow/6(ObjectID)
  ObjMovState/1 -> TOS_ObjMovStateCfmFlow/5(ObjMovState)
  ACC_Target_MovState_K2/1 -> TOS_ObjMovStateCfmFlow/4(Target_MovState_K2)
  ACC_Target_MovState_K1/1 -> TOS_ObjMovStateCfmFlow/3(Target_MovState_K1)
  ACC_Target_ID_K2/1 -> TOS_ObjMovStateCfmFlow/2(Target_ID_K2)
  ACC_Target_ID_K1/1 -> TOS_ObjMovStateCfmFlow/1(Target_ID_K1)
  TOS_ObjMovStateCfmFlow/1(TOS_ObjMovStateCfm) -> TOS_ObjMovStateCfm/1

== system PubIfDecisionTOS_MDL/TOS_20201112/TOS_2012080320/TOS/ACC/TOS_ACCCurrentLane/ACC_CurrentLane_Target/TOS_ACC_P1/ACC_P1_Targe/ACC_P1_Targe/TOS_ACC_TargetMovingDirConfirm/TOS_ACCMovingDirAborDly ==
  ACC_TargetP0_ID_K1 : Inport
  ObjectID : Inport  Port=2
  TOS_ACCMovingDir : Inport  Port=3
  If : If  IfExpression=u1
  If Action Subsystem : Subsystem  TreatAsAtomicUnit=on
  If Action Subsystem1 : Subsystem  TreatAsAtomicUnit=on
  Merge : Merge
  Subsystem : Subsystem
  TOS_ACC_TrgMovDirFlag_6_ObserVale : Outport
  TOS_ACC_TrgMovDir : Outport  Port=2
  wires:
  Merge/1 -> TOS_ACC_TrgMovDir/1
  If Action Subsystem/1(TOS_ACCMovingDirFilt) -> Merge/2
  If Action Subsystem1/1(TOS_ACCMovingDirFilt) -> Merge/1
  Subsystem/1(ACC_SameTargetP0) -> If/1, TOS_ACC_TrgMovDirFlag_6_ObserVale/1
  ObjectID/1 -> Subsystem/2(ObjectID)
  ACC_TargetP0_ID_K1/1 -> Subsystem/1(ACC_TargetP0_ID_K1)
  If/2 -> If Action Subsystem/Action
  TOS_ACCMovingDir/1 -> If Action Subsystem/1(TOS_ACCMovingDir), If Action Subsystem1/1(TOS_ACCMovingDir)
  If/1 -> If Action Subsystem1/Action

== system PubIfDecisionTOS_MDL/TOS_20201112/TOS_2012080320/TOS/ACC/TOS_ACCLeftLane/ACC_LeftLane_Target/TOS_ACC_P2/ACC_P2_Targe/ACC_P2_Targe/TOS_ACC_FusionTypeConfirm/Subsystem1 ==
  ObjMovState : Inport
  ACC_Target_ID_K1 : Inport  Port=2
  ACC_Target_ID_K2 : Inport  Port=3
  ACC_Target_MovState_K1 : Inport  Port=4
  ACC_Target_MovState_K2 : Inport  Port=5
  ObjectID : Inport  Port=6
  TOS_ObjMovStateCfmFlow1 : Stateflow chart  TreatAsAtomicUnit=on
  TOS_ObjMovStateCfm : Outport
  wires:
  ObjectID/1 -> TOS_ObjMovStateCfmFlow1/6(ObjectID)
  ObjMovState/1 -> TOS_ObjMovStateCfmFlow1/5(ObjMovState)
  ACC_Target_MovState_K2/1 -> TOS_ObjMovStateCfmFlow1/4(Target_MovState_K2)
  ACC_Target_MovState_K1/1 -> TOS_ObjMovStateCfmFlow1/3(Target_MovState_K1)
  ACC_Target_ID_K2/1 -> TOS_ObjMovStateCfmFlow1/2(Target_ID_K2)
  ACC_Target_ID_K1/1 -> TOS_ObjMovStateCfmFlow1/1(Target_ID_K1)
  TOS_ObjMovStateCfmFlow1/1(TOS_ObjMovStateCfm) -> TOS_ObjMovStateCfm/1

== system PubIfDecisionTOS_MDL/TOS_20201112/TOS_2012080320/TOS/ACC/TOS_ACCLeftLane/ACC_LeftLane_Target/TOS_ACC_P2/ACC_P2_Targe/ACC_P2_Targe/TOS_ACC_FusionTypeConfirm/TOS_ACCFusionTypeAborDly ==
  ACC_TargetP0_ID_K1 : Inport
  ObjectID : Inport  Port=2
  TOS_ACCFusionType : Inport  Port=3
  If : If  IfExpression=u1
  If Action Subsystem : Subsystem  TreatAsAtomicUnit=on
  If Action Subsystem1 : Subsystem  TreatAsAtomicUnit=on
  Merge : Merge
  Relational Operator : RelationalOperator  Operator===  OutDataTypeStr=boolean  RndMeth=Simplest
  TOS_ACCFusionTypeFilt : Outport
  wires:
  Merge/1 -> TOS_ACCFusionTypeFilt/1
  If Action Subsystem/1(TOS_ACCFusionTypeFilt) -> Merge/2
  If Action Subsystem1/1(TOS_ACCFusionTypeFilt) -> Merge/1
  Relational Operator/1 -> If/1
  ObjectID/1 -> Relational Operator/2
  ACC_TargetP0_ID_K1/1 -> Relational Operator/1
  If/2 -> If Action Subsystem/Action
  TOS_ACCFusionType/1 -> If Action Subsystem/1(TOS_ACCFusionType), If Action Subsystem1/1(TOS_ACCFusionType)
  If/1 -> If Action Subsystem1/Action

== system PubIfDecisionTOS_MDL/TOS_20201112/TOS_2012080320/TOS/ACC/TOS_ACCLeftLane/ACC_LeftLane_Target/TOS_ACC_P2/ACC_P2_Targe/ACC_P2_Targe/TOS_ACC_ObjTypeConfirm/Subsystem1 ==
  note: 针对有选中的运动目标，运动状态突变为静止，改变其运动状态为运动
  object_MovingState : Inport
  ACC_Target_ID_K1 : Inport  Port=2
  ACC_Target_ID_K2 : Inport  Port=3
  ACC_Target_MovState_K1 : Inport  Port=4
  ACC_Target_MovState_K2 : Inport  Port=5
  ObjectID : Inport  Port=6
  Object_Type : Inport  Port=7
  Compare To Constant11 : simulink/Logic and Bit Operations/Compare To Constant  relop===  const=1  OutDataTypeStr=boolean
  Compare To Constant2 : simulink/Logic and Bit Operations/Compare To Constant  relop===  const=OFM_OBJ_MOVINGSTATE_E.MOVING  OutDataTypeStr=boolean
      settings: AttributesFormatString=OFM_OBJ_MOVINGSTATE_E.MOVING = 2
  Compare To Constant3 : simulink/Logic and Bit Operations/Compare To Constant  relop===  const=OFM_OBJ_MOVINGSTATE_E.MOVING_SLOWLY  OutDataTypeStr=boolean
      settings: AttributesFormatString=OFM_OBJ_MOVINGSTATE_E.MOVING_SLOWLY = 5
  Compare To Constant6 : simulink/Logic and Bit Operations/Compare To Constant  relop===  const=OFM_OBJ_MOVINGSTATE_E.STOPPED  OutDataTypeStr=boolean
      settings: AttributesFormatString=OFM_OBJ_MOVINGSTATE_E.STOPPED = 4
  Compare To Constant8 : simulink/Logic and Bit Operations/Compare To Constant  relop===  const=OFM_OBJ_TYPE_E.UNKNOWN_TYPE  OutDataTypeStr=boolean
      settings: AttributesFormatString=OFM_OBJ_TYPE_E.UNKNOWN_TYPE = 1
  Data Type Conversion2 : DataTypeConversion  OutDataTypeStr=Enum: OFM_OBJ_MOVINGSTATE_E
  Logical Operator : Logic  AllPortsSameDT=off  OutDataTypeStr=boolean
  Logical Operator2 : Logic  Operator=OR  Inputs=4  AllPortsSameDT=off  OutDataTypeStr=boolean
  Subsystem : Subsystem
  Output : Outport
  wires:
  ACC_Target_MovState_K2/1 -> Subsystem/5(ACC_Target_MovState_K2)
  Subsystem/1(TOS_ObjMovStateCfm) -> Compare To Constant11/1
  Data Type Conversion2/1 -> Compare To Constant2/1, Compare To Constant3/1, Compare To Constant6/1, Subsystem/1(ObjMovState)
  ObjectID/1 -> [ObjectID], Subsystem/6(ObjectID)
  ACC_Target_ID_K1/1 -> Subsystem/2(ACC_Target_ID_K1), [ACC_Target_ID_K1]
  Compare To Constant11/1 -> Logical Operator2/4
  Logical Operator2/1 -> Logical Operator/1
  ACC_Target_MovState_K1/1 -> Subsystem/4(ACC_Target_MovState_K1)
  Compare To Constant2/1 -> Logical Operator2/1
  Compare To Constant3/1 -> Logical Operator2/2
  Compare To Constant8/1 -> Logical Operator/2
  ACC_Target_ID_K2/1 -> Subsystem/3(ACC_Target_ID_K2)
  object_MovingState/1 -> Data Type Conversion2/1
  Compare To Constant6/1 -> Logical Operator2/3
  Object_Type/1 -> Compare To Constant8/1
  Logical Operator/1 -> Output/1

== system PubIfDecisionTOS_MDL/TOS_20201112/TOS_2012080320/TOS/ACC/TOS_ACCLeftLane/ACC_LeftLane_Target/TOS_ACC_P2/ACC_P2_Targe/ACC_P2_Targe/TOS_ACC_ObjTypeConfirm/TOS_ACCObjTypeAborDly ==
  ACC_Target_ID_K1 : Inport
  ObjectID : Inport  Port=2
  TOS_ACCObjType : Inport  Port=3
  If : If  IfExpression=u1
  If Action Subsystem : Subsystem  TreatAsAtomicUnit=on
  If Action Subsystem1 : Subsystem  TreatAsAtomicUnit=on
  Merge : Merge
  Relational Operator : RelationalOperator  Operator===  OutDataTypeStr=boolean  RndMeth=Simplest
  TOS_ACCObjTypeFilt : Outport
  wires:
  Merge/1 -> TOS_ACCObjTypeFilt/1
  If Action Subsystem/1(TOS_ACCFusionTypeFilt) -> Merge/2
  If Action Subsystem1/1(TOS_ACCFusionTypeFilt) -> Merge/1
  Relational Operator/1 -> If/1
  ObjectID/1 -> Relational Operator/2
  ACC_Target_ID_K1/1 -> Relational Operator/1
  If/2 -> If Action Subsystem/Action
  TOS_ACCObjType/1 -> If Action Subsystem/1(TOS_ACCFusionType), If Action Subsystem1/1(TOS_ACCFusionType)
  If/1 -> If Action Subsystem1/Action

== system PubIfDecisionTOS_MDL/TOS_20201112/TOS_2012080320/TOS/ACC/TOS_ACCLeftLane/ACC_LeftLane_Target/TOS_ACC_P2/ACC_P2_Targe/ACC_P2_Targe/TOS_ACC_ObstacleProbConfirm/TOS_ACCObstacleProbAborDly ==
  ACC_Target_ID_K1 : Inport
  ObjectID : Inport  Port=2
  TOS_ACCObstacleProb : Inport  Port=3
  If : If  IfExpression=u1
  If Action Subsystem : Subsystem  TreatAsAtomicUnit=on
  If Action Subsystem1 : Subsystem  TreatAsAtomicUnit=on
  Merge : Merge
  Subsystem : Subsystem
  TOS_ACCObstacleProbFilt : Outport
  wires:
  Merge/1 -> TOS_ACCObstacleProbFilt/1
  If Action Subsystem/1(TOS_ACCFusionTypeFilt) -> Merge/2
  If Action Subsystem1/1(TOS_ACCFusionTypeFilt) -> Merge/1
  Subsystem/1(ACC_SameTargetP0) -> If/1
  ObjectID/1 -> Subsystem/2(ObjectID)
  ACC_Target_ID_K1/1 -> Subsystem/1(ACC_TargetP0_ID_K1)
  If/2 -> If Action Subsystem/Action
  TOS_ACCObstacleProb/1 -> If Action Subsystem/1(TOS_ACCFusionType), If Action Subsystem1/1(TOS_ACCFusionType)
  If/1 -> If Action Subsystem1/Action

== system PubIfDecisionTOS_MDL/TOS_20201112/TOS_2012080320/TOS/ACC/TOS_ACCLeftLane/ACC_LeftLane_Target/TOS_ACC_P2/ACC_P2_Targe/ACC_P2_Targe/TOS_ACC_TargetMovingDirConfirm/Subsystem ==
  ObjMovState : Inport
  ACC_Target_ID_K1 : Inport  Port=2
  ACC_Target_ID_K2 : Inport  Port=3
  ACC_Target_MovState_K1 : Inport  Port=4
  ACC_Target_MovState_K2 : Inport  Port=5
  ObjectID : Inport  Port=6
  TOS_ObjMovStateCfmFlow : Stateflow chart  TreatAsAtomicUnit=on
  TOS_ObjMovStateCfm : Outport
  wires:
  ObjectID/1 -> TOS_ObjMovStateCfmFlow/6(ObjectID)
  ObjMovState/1 -> TOS_ObjMovStateCfmFlow/5(ObjMovState)
  ACC_Target_MovState_K2/1 -> TOS_ObjMovStateCfmFlow/4(Target_MovState_K2)
  ACC_Target_MovState_K1/1 -> TOS_ObjMovStateCfmFlow/3(Target_MovState_K1)
  ACC_Target_ID_K2/1 -> TOS_ObjMovStateCfmFlow/2(Target_ID_K2)
  ACC_Target_ID_K1/1 -> TOS_ObjMovStateCfmFlow/1(Target_ID_K1)
  TOS_ObjMovStateCfmFlow/1(TOS_ObjMovStateCfm) -> TOS_ObjMovStateCfm/1

== system PubIfDecisionTOS_MDL/TOS_20201112/TOS_2012080320/TOS/ACC/TOS_ACCLeftLane/ACC_LeftLane_Target/TOS_ACC_P2/ACC_P2_Targe/ACC_P2_Targe/TOS_ACC_TargetMovingDirConfirm/TOS_ACCMovingDirAborDly ==
  ACC_TargetP0_ID_K1 : Inport
  ObjectID : Inport  Port=2
  TOS_ACCMovingDir : Inport  Port=3
  If : If  IfExpression=u1
  If Action Subsystem : Subsystem  TreatAsAtomicUnit=on
  If Action Subsystem1 : Subsystem  TreatAsAtomicUnit=on
  Merge : Merge
  Subsystem : Subsystem
  TOS_ACC_TrgMovDirFlag_6_ObserVale : Outport
  TOS_ACC_TrgMovDir : Outport  Port=2
  wires:
  Merge/1 -> TOS_ACC_TrgMovDir/1
  If Action Subsystem/1(TOS_ACCMovingDirFilt) -> Merge/2
  If Action Subsystem1/1(TOS_ACCMovingDirFilt) -> Merge/1
  Subsystem/1(ACC_SameTargetP0) -> If/1, TOS_ACC_TrgMovDirFlag_6_ObserVale/1
  ObjectID/1 -> Subsystem/2(ObjectID)
  ACC_TargetP0_ID_K1/1 -> Subsystem/1(ACC_TargetP0_ID_K1)
  If/2 -> If Action Subsystem/Action
  TOS_ACCMovingDir/1 -> If Action Subsystem/1(TOS_ACCMovingDir), If Action Subsystem1/1(TOS_ACCMovingDir)
  If/1 -> If Action Subsystem1/Action

== system PubIfDecisionTOS_MDL/TOS_20201112/TOS_2012080320/TOS/ACC/TOS_ACCLeftLane/ACC_LeftLane_Target/TOS_ACC_P4/ACC_P4_Targe/ACC_P4_Targe/TOS_ACC_FusionTypeConfirm/Subsystem1 ==
  ObjMovState : Inport
  ACC_Target_ID_K1 : Inport  Port=2
  ACC_Target_ID_K2 : Inport  Port=3
  ACC_Target_MovState_K1 : Inport  Port=4
  ACC_Target_MovState_K2 : Inport  Port=5
  ObjectID : Inport  Port=6
  TOS_ObjMovStateCfmFlow1 : Stateflow chart  TreatAsAtomicUnit=on
  TOS_ObjMovStateCfm : Outport
  wires:
  TOS_ObjMovStateCfmFlow1/1(TOS_ObjMovStateCfm) -> TOS_ObjMovStateCfm/1
  ACC_Target_ID_K1/1 -> TOS_ObjMovStateCfmFlow1/1(Target_ID_K1)
  ACC_Target_ID_K2/1 -> TOS_ObjMovStateCfmFlow1/2(Target_ID_K2)
  ACC_Target_MovState_K1/1 -> TOS_ObjMovStateCfmFlow1/3(Target_MovState_K1)
  ACC_Target_MovState_K2/1 -> TOS_ObjMovStateCfmFlow1/4(Target_MovState_K2)
  ObjMovState/1 -> TOS_ObjMovStateCfmFlow1/5(ObjMovState)
  ObjectID/1 -> TOS_ObjMovStateCfmFlow1/6(ObjectID)

== system PubIfDecisionTOS_MDL/TOS_20201112/TOS_2012080320/TOS/ACC/TOS_ACCLeftLane/ACC_LeftLane_Target/TOS_ACC_P4/ACC_P4_Targe/ACC_P4_Targe/TOS_ACC_FusionTypeConfirm/TOS_ACCFusionTypeAborDly ==
  ACC_TargetP0_ID_K1 : Inport
  ObjectID : Inport  Port=2
  TOS_ACCFusionType : Inport  Port=3
  If : If  IfExpression=u1
  If Action Subsystem : Subsystem  TreatAsAtomicUnit=on
  If Action Subsystem1 : Subsystem  TreatAsAtomicUnit=on
  Merge : Merge
  Relational Operator : RelationalOperator  Operator===  OutDataTypeStr=boolean  RndMeth=Simplest
  TOS_ACCFusionTypeFilt : Outport
  wires:
  If/1 -> If Action Subsystem1/Action
  TOS_ACCFusionType/1 -> If Action Subsystem1/1(TOS_ACCFusionType), If Action Subsystem/1(TOS_ACCFusionType)
  If/2 -> If Action Subsystem/Action
  ACC_TargetP0_ID_K1/1 -> Relational Operator/1
  ObjectID/1 -> Relational Operator/2
  Relational Operator/1 -> If/1
  If Action Subsystem1/1(TOS_ACCFusionTypeFilt) -> Merge/1
  If Action Subsystem/1(TOS_ACCFusionTypeFilt) -> Merge/2
  Merge/1 -> TOS_ACCFusionTypeFilt/1

== system PubIfDecisionTOS_MDL/TOS_20201112/TOS_2012080320/TOS/ACC/TOS_ACCLeftLane/ACC_LeftLane_Target/TOS_ACC_P4/ACC_P4_Targe/ACC_P4_Targe/TOS_ACC_ObjTypeConfirm/Subsystem1 ==
  note: 针对有选中的运动目标，运动状态突变为静止，改变其运动状态为运动
  object_MovingState : Inport
  ACC_Target_ID_K1 : Inport  Port=2
  ACC_Target_ID_K2 : Inport  Port=3
  ACC_Target_MovState_K1 : Inport  Port=4
  ACC_Target_MovState_K2 : Inport  Port=5
  ObjectID : Inport  Port=6
  Object_Type : Inport  Port=7
  Compare To Constant11 : simulink/Logic and Bit Operations/Compare To Constant  relop===  const=1  OutDataTypeStr=boolean
  Compare To Constant2 : simulink/Logic and Bit Operations/Compare To Constant  relop===  const=OFM_OBJ_MOVINGSTATE_E.MOVING  OutDataTypeStr=boolean
      settings: AttributesFormatString=OFM_OBJ_MOVINGSTATE_E.MOVING = 2
  Compare To Constant3 : simulink/Logic and Bit Operations/Compare To Constant  relop===  const=OFM_OBJ_MOVINGSTATE_E.MOVING_SLOWLY  OutDataTypeStr=boolean
      settings: AttributesFormatString=OFM_OBJ_MOVINGSTATE_E.MOVING_SLOWLY = 5
  Compare To Constant6 : simulink/Logic and Bit Operations/Compare To Constant  relop===  const=OFM_OBJ_MOVINGSTATE_E.STOPPED  OutDataTypeStr=boolean
      settings: AttributesFormatString=OFM_OBJ_MOVINGSTATE_E.STOPPED = 4
  Compare To Constant8 : simulink/Logic and Bit Operations/Compare To Constant  relop===  const=OFM_OBJ_TYPE_E.UNKNOWN_TYPE  OutDataTypeStr=boolean
      settings: AttributesFormatString=OFM_OBJ_TYPE_E.UNKNOWN_TYPE = 1
  Data Type Conversion2 : DataTypeConversion  OutDataTypeStr=Enum: OFM_OBJ_MOVINGSTATE_E
  Logical Operator : Logic  AllPortsSameDT=off  OutDataTypeStr=boolean
  Logical Operator2 : Logic  Operator=OR  Inputs=4  AllPortsSameDT=off  OutDataTypeStr=boolean
  Subsystem : Subsystem
  Output : Outport
  wires:
  Logical Operator/1 -> Output/1
  Object_Type/1 -> Compare To Constant8/1
  Compare To Constant6/1 -> Logical Operator2/3
  object_MovingState/1 -> Data Type Conversion2/1
  ACC_Target_ID_K2/1 -> Subsystem/3(ACC_Target_ID_K2)
  Compare To Constant8/1 -> Logical Operator/2
  Compare To Constant3/1 -> Logical Operator2/2
  Compare To Constant2/1 -> Logical Operator2/1
  ACC_Target_MovState_K1/1 -> Subsystem/4(ACC_Target_MovState_K1)
  Logical Operator2/1 -> Logical Operator/1
  Compare To Constant11/1 -> Logical Operator2/4
  ACC_Target_ID_K1/1 -> [ACC_Target_ID_K1], Subsystem/2(ACC_Target_ID_K1)
  ObjectID/1 -> Subsystem/6(ObjectID), [ObjectID]
  Data Type Conversion2/1 -> Subsystem/1(ObjMovState), Compare To Constant6/1, Compare To Constant3/1, Compare To Constant2/1
  Subsystem/1(TOS_ObjMovStateCfm) -> Compare To Constant11/1
  ACC_Target_MovState_K2/1 -> Subsystem/5(ACC_Target_MovState_K2)

== system PubIfDecisionTOS_MDL/TOS_20201112/TOS_2012080320/TOS/ACC/TOS_ACCLeftLane/ACC_LeftLane_Target/TOS_ACC_P4/ACC_P4_Targe/ACC_P4_Targe/TOS_ACC_ObjTypeConfirm/TOS_ACCObjTypeAborDly ==
  ACC_Target_ID_K1 : Inport
  ObjectID : Inport  Port=2
  TOS_ACCObjType : Inport  Port=3
  If : If  IfExpression=u1
  If Action Subsystem : Subsystem  TreatAsAtomicUnit=on
  If Action Subsystem1 : Subsystem  TreatAsAtomicUnit=on
  Merge : Merge
  Relational Operator : RelationalOperator  Operator===  OutDataTypeStr=boolean  RndMeth=Simplest
  TOS_ACCObjTypeFilt : Outport
  wires:
  If/1 -> If Action Subsystem1/Action
  TOS_ACCObjType/1 -> If Action Subsystem1/1(TOS_ACCFusionType), If Action Subsystem/1(TOS_ACCFusionType)
  If/2 -> If Action Subsystem/Action
  ACC_Target_ID_K1/1 -> Relational Operator/1
  ObjectID/1 -> Relational Operator/2
  Relational Operator/1 -> If/1
  If Action Subsystem1/1(TOS_ACCFusionTypeFilt) -> Merge/1
  If Action Subsystem/1(TOS_ACCFusionTypeFilt) -> Merge/2
  Merge/1 -> TOS_ACCObjTypeFilt/1

== system PubIfDecisionTOS_MDL/TOS_20201112/TOS_2012080320/TOS/ACC/TOS_ACCLeftLane/ACC_LeftLane_Target/TOS_ACC_P4/ACC_P4_Targe/ACC_P4_Targe/TOS_ACC_ObstacleProbConfirm/TOS_ACCObstacleProbAborDly ==
  ACC_Target_ID_K1 : Inport
  ObjectID : Inport  Port=2
  TOS_ACCObstacleProb : Inport  Port=3
  If : If  IfExpression=u1
  If Action Subsystem : Subsystem  TreatAsAtomicUnit=on
  If Action Subsystem1 : Subsystem  TreatAsAtomicUnit=on
  Merge : Merge
  Subsystem : Subsystem
  TOS_ACCObstacleProbFilt : Outport
  wires:
  If/1 -> If Action Subsystem1/Action
  TOS_ACCObstacleProb/1 -> If Action Subsystem1/1(TOS_ACCFusionType), If Action Subsystem/1(TOS_ACCFusionType)
  If/2 -> If Action Subsystem/Action
  ACC_Target_ID_K1/1 -> Subsystem/1(ACC_TargetP0_ID_K1)
  ObjectID/1 -> Subsystem/2(ObjectID)
  Subsystem/1(ACC_SameTargetP0) -> If/1
  If Action Subsystem1/1(TOS_ACCFusionTypeFilt) -> Merge/1
  If Action Subsystem/1(TOS_ACCFusionTypeFilt) -> Merge/2
  Merge/1 -> TOS_ACCObstacleProbFilt/1

== system PubIfDecisionTOS_MDL/TOS_20201112/TOS_2012080320/TOS/ACC/TOS_ACCLeftLane/ACC_LeftLane_Target/TOS_ACC_P4/ACC_P4_Targe/ACC_P4_Targe/TOS_ACC_TargetMovingDirConfirm/Subsystem ==
  ObjMovState : Inport
  ACC_Target_ID_K1 : Inport  Port=2
  ACC_Target_ID_K2 : Inport  Port=3
  ACC_Target_MovState_K1 : Inport  Port=4
  ACC_Target_MovState_K2 : Inport  Port=5
  ObjectID : Inport  Port=6
  TOS_ObjMovStateCfmFlow : Stateflow chart  TreatAsAtomicUnit=on
  TOS_ObjMovStateCfm : Outport
  wires:
  TOS_ObjMovStateCfmFlow/1(TOS_ObjMovStateCfm) -> TOS_ObjMovStateCfm/1
  ACC_Target_ID_K1/1 -> TOS_ObjMovStateCfmFlow/1(Target_ID_K1)
  ACC_Target_ID_K2/1 -> TOS_ObjMovStateCfmFlow/2(Target_ID_K2)
  ACC_Target_MovState_K1/1 -> TOS_ObjMovStateCfmFlow/3(Target_MovState_K1)
  ACC_Target_MovState_K2/1 -> TOS_ObjMovStateCfmFlow/4(Target_MovState_K2)
  ObjMovState/1 -> TOS_ObjMovStateCfmFlow/5(ObjMovState)
  ObjectID/1 -> TOS_ObjMovStateCfmFlow/6(ObjectID)

== system PubIfDecisionTOS_MDL/TOS_20201112/TOS_2012080320/TOS/ACC/TOS_ACCLeftLane/ACC_LeftLane_Target/TOS_ACC_P4/ACC_P4_Targe/ACC_P4_Targe/TOS_ACC_TargetMovingDirConfirm/TOS_ACCMovingDirAborDly ==
  ACC_TargetP0_ID_K1 : Inport
  ObjectID : Inport  Port=2
  TOS_ACCMovingDir : Inport  Port=3
  If : If  IfExpression=u1
  If Action Subsystem : Subsystem  TreatAsAtomicUnit=on
  If Action Subsystem1 : Subsystem  TreatAsAtomicUnit=on
  Merge : Merge
  Subsystem : Subsystem
  TOS_ACC_TrgMovDirFlag_6_ObserVale : Outport
  TOS_ACC_TrgMovDir : Outport  Port=2
  wires:
  If/1 -> If Action Subsystem1/Action
  TOS_ACCMovingDir/1 -> If Action Subsystem1/1(TOS_ACCMovingDir), If Action Subsystem/1(TOS_ACCMovingDir)
  If/2 -> If Action Subsystem/Action
  ACC_TargetP0_ID_K1/1 -> Subsystem/1(ACC_TargetP0_ID_K1)
  ObjectID/1 -> Subsystem/2(ObjectID)
  Subsystem/1(ACC_SameTargetP0) -> TOS_ACC_TrgMovDirFlag_6_ObserVale/1, If/1
  If Action Subsystem1/1(TOS_ACCMovingDirFilt) -> Merge/1
  If Action Subsystem/1(TOS_ACCMovingDirFilt) -> Merge/2
  Merge/1 -> TOS_ACC_TrgMovDir/1

== system PubIfDecisionTOS_MDL/TOS_20201112/TOS_2012080320/TOS/ACC/TOS_ACCRightLane/ACC_LeftLane_Target/TOS_ACC_P3/ACC_P3_Targe/ACC_P3_Targe/TOS_ACC_FusionTypeConfirm/Subsystem1 ==
  ObjMovState : Inport
  ACC_Target_ID_K1 : Inport  Port=2
  ACC_Target_ID_K2 : Inport  Port=3
  ACC_Target_MovState_K1 : Inport  Port=4
  ACC_Target_MovState_K2 : Inport  Port=5
  ObjectID : Inport  Port=6
  TOS_ObjMovStateCfmFlow1 : Stateflow chart  TreatAsAtomicUnit=on
  TOS_ObjMovStateCfm : Outport
  wires:
  ObjectID/1 -> TOS_ObjMovStateCfmFlow1/6(ObjectID)
  ObjMovState/1 -> TOS_ObjMovStateCfmFlow1/5(ObjMovState)
  ACC_Target_MovState_K2/1 -> TOS_ObjMovStateCfmFlow1/4(Target_MovState_K2)
  ACC_Target_MovState_K1/1 -> TOS_ObjMovStateCfmFlow1/3(Target_MovState_K1)
  ACC_Target_ID_K2/1 -> TOS_ObjMovStateCfmFlow1/2(Target_ID_K2)
  ACC_Target_ID_K1/1 -> TOS_ObjMovStateCfmFlow1/1(Target_ID_K1)
  TOS_ObjMovStateCfmFlow1/1(TOS_ObjMovStateCfm) -> TOS_ObjMovStateCfm/1

== system PubIfDecisionTOS_MDL/TOS_20201112/TOS_2012080320/TOS/ACC/TOS_ACCRightLane/ACC_LeftLane_Target/TOS_ACC_P3/ACC_P3_Targe/ACC_P3_Targe/TOS_ACC_FusionTypeConfirm/TOS_ACCFusionTypeAborDly ==
  ACC_TargetP0_ID_K1 : Inport
  ObjectID : Inport  Port=2
  TOS_ACCFusionType : Inport  Port=3
  If : If  IfExpression=u1
  If Action Subsystem : Subsystem  TreatAsAtomicUnit=on
  If Action Subsystem1 : Subsystem  TreatAsAtomicUnit=on
  Merge : Merge
  Relational Operator : RelationalOperator  Operator===  OutDataTypeStr=boolean  RndMeth=Simplest
  TOS_ACCFusionTypeFilt : Outport
  wires:
  Merge/1 -> TOS_ACCFusionTypeFilt/1
  If Action Subsystem/1(TOS_ACCFusionTypeFilt) -> Merge/2
  If Action Subsystem1/1(TOS_ACCFusionTypeFilt) -> Merge/1
  Relational Operator/1 -> If/1
  ObjectID/1 -> Relational Operator/2
  ACC_TargetP0_ID_K1/1 -> Relational Operator/1
  If/2 -> If Action Subsystem/Action
  TOS_ACCFusionType/1 -> If Action Subsystem/1(TOS_ACCFusionType), If Action Subsystem1/1(TOS_ACCFusionType)
  If/1 -> If Action Subsystem1/Action
